simulink model "model1_StateEstimator"  (R2020a)
settings: Solver=FixedStepAuto  StartTime=0.0  StopTime=T  FixedStep=Ts  RelTol=1e-3
undefined symbols (not defined in the file): L, Lb, Ts, wn, x0, zeta
settings Model: Creator=XiaoCY  LastModifiedBy=XiaoCY
settings DataIOCC: ReturnWorkspaceOutputs=off

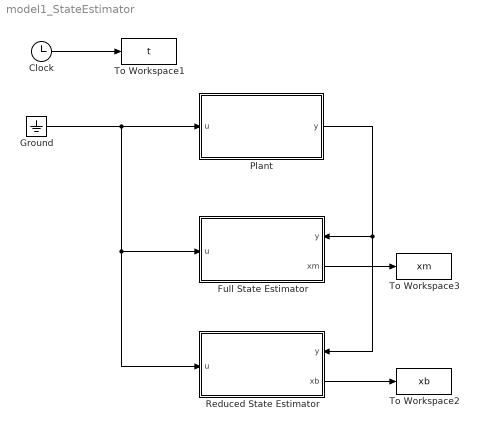
== system model1_StateEstimator ==
  Clock : Clock
  Full State Estimator : Subsystem
      settings: PortSchema="{\"entries\":[{\"content\":{\"sides\":[{\"content\":{\"connectorIds\":[\"In1\"]},\"type\":\"ConnectorPlacement.EquallySpacedRectSide\",\"uuid\":\"e2a857a4-4215-476a-958a-7445ed69b3c3\"},{\"content\":{\"connectorIds\":[\"In2\",\"Out1\"],\"side\":\"RIGHT\"},\"type\":\"ConnectorPlacement.EquallySpacedRectSide\",\"uuid\":\"f40b62ad-c08a-46ea-a3b8-aa7694558cdb\"},{\"content\":{\"connectorIds\":[],\"side\":\"TOP\"},\"type\":\"ConnectorPlacement.EquallySpacedRectSide\",\"uuid\":\"4b61a7e3-43b7-4a5d-a93a-c25485f178a0\"}]},\"type\":\"ConnectorPlacement.EquallySpacedConnector\",\"uuid\":\"82723d51-c1ed-49c7-81a4-0fd477216f4d\"}],\"packageUris\":[\"http://schema.mathworks.com/mf0/Connector/19700101\"],\"version\":\"1.0\"}"
  Ground : Ground
  Plant : Subsystem
  Reduced State Estimator : Subsystem
      settings: PortSchema="{\"entries\":[{\"content\":{\"sides\":[{\"content\":{\"connectorIds\":[\"In1\"]},\"type\":\"ConnectorPlacement.EquallySpacedRectSide\",\"uuid\":\"e2a857a4-4215-476a-958a-7445ed69b3c3\"},{\"content\":{\"connectorIds\":[\"In2\",\"Out1\"],\"side\":\"RIGHT\"},\"type\":\"ConnectorPlacement.EquallySpacedRectSide\",\"uuid\":\"f40b62ad-c08a-46ea-a3b8-aa7694558cdb\"},{\"content\":{\"connectorIds\":[],\"side\":\"TOP\"},\"type\":\"ConnectorPlacement.EquallySpacedRectSide\",\"uuid\":\"4b61a7e3-43b7-4a5d-a93a-c25485f178a0\"}]},\"type\":\"ConnectorPlacement.EquallySpacedConnector\",\"uuid\":\"82723d51-c1ed-49c7-81a4-0fd477216f4d\"}],\"packageUris\":[\"http://schema.mathworks.com/mf0/Connector/19700101\"],\"version\":\"1.0\"}"
  To Workspace1 : ToWorkspace  VariableName=t  SampleTime=Ts
  To Workspace2 : ToWorkspace  VariableName=xb  SampleTime=Ts
  To Workspace3 : ToWorkspace  VariableName=xm  SampleTime=Ts
  wires:
  Clock/1 -> To Workspace1/1
  Plant/1(y) -> Reduced State Estimator/2(y), Full State Estimator/2(y)
  Full State Estimator/1(xm) -> To Workspace3/1
  Ground/1 -> Reduced State Estimator/1(u), Full State Estimator/1(u), Plant/1(u)
  Reduced State Estimator/1(xb) -> To Workspace2/1

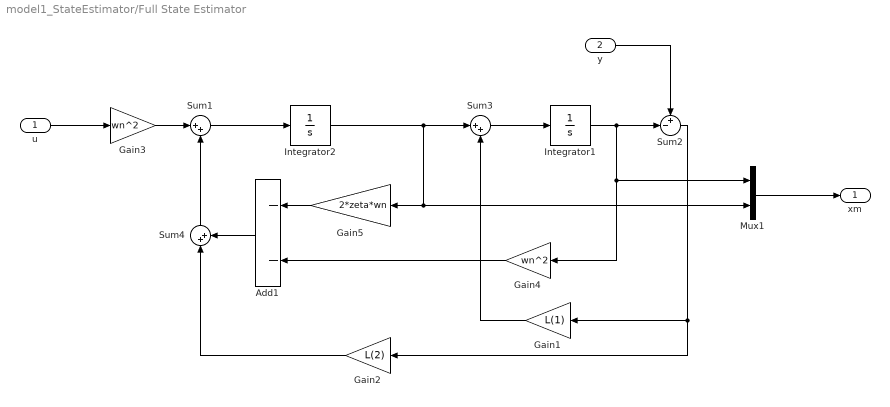
== system model1_StateEstimator/Full State Estimator ==
  u : Inport
  y : Inport  Port=2
  Add1 : Sum  Inputs=--
  Gain1 : Gain  Gain=L(1)
  Gain2 : Gain  Gain=L(2)
  Gain3 : Gain  Gain=wn^2
  Gain4 : Gain  Gain=wn^2
  Gain5 : Gain  Gain=2*zeta*wn
  Integrator1 : Integrator
  Integrator2 : Integrator
  Mux1 : Mux  Inputs=2
  Sum1 : Sum  Inputs=|++
  Sum2 : Sum  Inputs=+-|
  Sum3 : Sum  Inputs=|++
  Sum4 : Sum  Inputs=|++
  xm : Outport
  wires:
  Mux1/1 -> xm/1
  Integrator2/1 -> Sum3/1, Gain5/1, Mux1/2
  Gain5/1 -> Add1/1
  Add1/1 -> Sum4/2
  Sum1/1 -> Integrator2/1
  Gain3/1 -> Sum1/1
  Integrator1/1 -> Gain4/1, Mux1/1, Sum2/2
  y/1 -> Sum2/1
  u/1 -> Gain3/1
  Sum2/1 -> Gain1/1, Gain2/1
  Sum3/1 -> Integrator1/1
  Gain2/1 -> Sum4/1
  Sum4/1 -> Sum1/2
  Gain4/1 -> Add1/2
  Gain1/1 -> Sum3/2

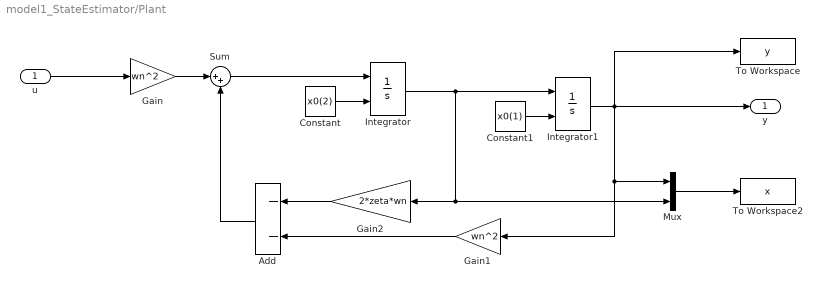
== system model1_StateEstimator/Plant ==
  u : Inport
  Add : Sum  Inputs=--
  Constant : Constant  Value=x0(2)
  Constant1 : Constant  Value=x0(1)
  Gain : Gain  Gain=wn^2
  Gain1 : Gain  Gain=wn^2
  Gain2 : Gain  Gain=2*zeta*wn
  Integrator : Integrator  InitialConditionSource=external
  Integrator1 : Integrator  InitialConditionSource=external
  Mux : Mux  Inputs=2
  Sum : Sum  Inputs=|++
  To Workspace : ToWorkspace  VariableName=y  SampleTime=Ts
  To Workspace2 : ToWorkspace  VariableName=x  SampleTime=Ts
  y : Outport
  wires:
  Integrator/1 -> Gain2/1, Mux/2, Integrator1/1
  Mux/1 -> To Workspace2/1
  Gain/1 -> Sum/1
  Integrator1/1 -> To Workspace/1, y/1, Mux/1, Gain1/1
  Constant/1 -> Integrator/2
  Sum/1 -> Integrator/1
  Gain1/1 -> Add/2
  Constant1/1 -> Integrator1/2
  Gain2/1 -> Add/1
  u/1 -> Gain/1
  Add/1 -> Sum/2

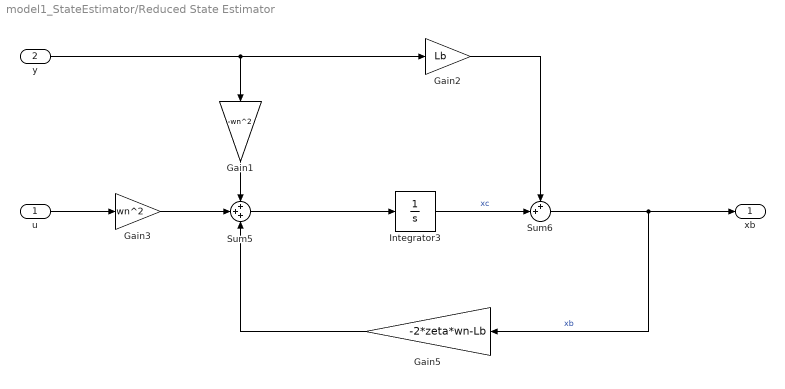
== system model1_StateEstimator/Reduced State Estimator ==
  u : Inport
  y : Inport  Port=2
  Gain1 : Gain  Gain=-wn^2
  Gain2 : Gain  Gain=Lb
  Gain3 : Gain  Gain=wn^2
  Gain5 : Gain  Gain=-2*zeta*wn-Lb
  Integrator3 : Integrator
  Sum5 : Sum  Inputs=+++
  Sum6 : Sum  Inputs=++|
  xb : Outport
  wires:
  Gain5/1 -> Sum5/3
  u/1 -> Gain3/1
  Sum5/1 -> Integrator3/1
  Integrator3/1 -> Sum6/2  "xc"
  Gain3/1 -> Sum5/2
  y/1 -> Gain2/1, Gain1/1
  Gain2/1 -> Sum6/1
  Sum6/1 -> Gain5/1, xb/1  "xb"
  Gain1/1 -> Sum5/1
